simulink model "RB_KAIROS_impControl_repulsive"  (R2020b)
settings: Solver=ode4  StartTime=0.0  StopTime=t_end  FixedStep=Ts  RelTol=1e-3
values from neighbouring files (symbols this model uses):
  am = 0.3    [RB_KAIROS_ImpControl_OpSpace_quat_2020b_safety_main.m]
  am_r = 0.3    [RB_KAIROS_ImpControl_OpSpace_quat_2020b_safety_main.m]
  Kc = diag(50*ones(6,1))    [RB_KAIROS_ImpControl_OpSpace_quat_2020b_safety_main.m]
  Kp = 2*[400;400;400;400;0;0;0]    [RB_KAIROS_ImpControl_OpSpace_quat_2020b_safety_main.m]
  Kv = [1000;1000;1000;[300;300;300;300;300;300;300]]    [RB_KAIROS_ImpControl_OpSpace_quat_2020b_safety_main.m]
  model_sample_time = 0.001    [RB_KAIROS_ImpControl_OpSpace_quat_2020b_safety_main.m]
  q_dot_0 = zeros(10,1)    [RB_KAIROS_ImpControl_OpSpace_quat_2020b_safety_main.m]
  T_i = K    [RB_KAIROS_ImpControl_OpSpace_quat_2020b_safety_main.m]
  tau_ext = [0 0 0 0 0 0 0 0 0 0 0]    [RB_KAIROS_ImpControl_OpSpace_quat_2020b_safety_main.m]
  v_SMU = 10    [RB_KAIROS_ImpControl_OpSpace_quat_2020b_safety_main.m]
  vm = 0.5    [RB_KAIROS_ImpControl_OpSpace_quat_2020b_safety_main.m]
  vm_r = 0.5    [RB_KAIROS_ImpControl_OpSpace_quat_2020b_safety_main.m]
undefined symbols (not defined in the file or in its folder): DiscIntNeverNeededParam, magnitude, q_0, T_f
libraries: simulink x4, utils x4, transformations_lib x3
(part 12 of 17)

== matlab function RB_KAIROS_impControl_repulsive/Trajectory Generator/move2pose/fs_function ==
  data: opti_break output; T_est output; Tm input; time_step input; t input; vc input; vd input; vm input; v_smu input; am input; Gamma input; Theta input; k input; T_scale input; time_factor output; interpoly input; rethink_point input; start_lvl input; stop_lvl input; reset input
function [opti_break,T_est,time_factor] = fs_function_time_rethink(Tm, time_step, t, vc, vd, vm, v_smu, am, Gamma, Theta, k, T_scale, interpoly, rethink_point, start_lvl, stop_lvl, reset)
%%% This function decides which version to call; Or when/if a rethink is
%%% done.
% 0 =       internship version (only with minor bugfixes)
% 1 and 2 = start with half the velocity, then rethink, then linear part and
%           rest is the original full half
% 3 =       general solution, heading to vd always (best option)
% 4 =       general solution, heading to v_smu if going down

time_factor = 0;
opti_break = 0;
T_est = 0;
psi  = psi_velocity(vm, vd);
switch rethink_point
    case 0
        time_factor = fs_function_time_f(t, T_scale, psi, Gamma, Theta, k, interpoly);
    case 1
        T = T_calc(vc,vd,vm,am,T_scale,interpoly);
        [time_factor,opti_break,T_est] = fs_function_time_hlf(Tm, t, T, psi, Gamma, Theta, k, interpoly, time_step);
    case 2
        [time_factor,opti_break,T_est] = fs_function_time_g(Tm, t, T_scale, psi, Gamma, Theta, k, interpoly, time_step, 0, 0.5, 3, vm, am, v_smu, reset);
    case 3
        [time_factor,opti_break,T_est] = fs_function_time_g(Tm, t, T_scale, psi, Gamma, Theta, k, interpoly, time_step, start_lvl, stop_lvl, rethink_point, vm, am, v_smu, reset);
    case 4
        [time_factor,opti_break,T_est] = fs_function_time_g(Tm, t, T_scale, psi, Gamma, Theta, k, interpoly, time_step, start_lvl, stop_lvl, rethink_point, vm, am, v_smu, reset);
    otherwise
        error('Unknown rethink_point');       %rest
end

end

function [time_factor,opti_break,T_est] = fs_function_time_g(Tm, t, T_scale, psi, Gamma, Theta, k, interpoly, time_step, start_lvl, stop_lvl, rethink_point, vm, am, v_smu, reset)
%FS_FUNCTION_TIME computes the scaling factor for the next timestep. The idea is 
% similar to equotation (14) of the reference. This is
% achieved by the introduction of time t and setting a duration T for the
% adaption.
%
% This is the most general solution so far. It accelerates till am and then
% it stays on this level till it has to decelerate again to reach the new
% velocity level. The velocity level could be updated in any timestep.
%
% Reference:
% [1] S. Haddadin, A. Albu-Schäffer, A. De Luca, and G. Hirzinger, 
% "Collision detection and reaction: A contribution to safe physical 
% human-robot interaction,” International Conference on Intelligent Robots 
% and Systems, pp. 3356–3363, 2008.
%
% Input variables
% Tm          = Maximum time left for adaption
% t           = Current runtime
% T_scale     = Scaling factor for duration of adaption
% psi         = Scaling factor for time
% Gamma       = Optional dead-zone between stop and reverting motion (set 0
%               for deactivation)
% Theta       = Optional smoothness or strechting(set 1 for deactivation) 
% k           = speed factor for pushing back; 1=deactivated; the higher 
%               the faster the reverting motion
% interpoly   = Which interpolation to use
% time_step   = Duration of one time step
% start_lvl   = percentage for delta_psi_start: [0;1[ (Do not set to near to one!)
% stop_lvl    = percentage for delta_psi_stop: [0;1[ (Do not set to near to one!)
% rethink_point
%             = choose on which velocity the percentage is used
% vm          = maximum allowed velocity
% am          = maximum allowed acceleration
% v_smu       = Real v_smu
% reset       = If this is one, the psi_1 variable is reseted; only needed
%               due to reversing motion
%
% Output variables
% time_factor = Factor for scaling the next time increment; 0=Stop motion;
%               1= Normal speed; negative values = revert motion
% opti_break  = Trigger for optimal breaking; is set to 1 if Tm<T_est
% T_est       = Current estimate of the duration of the adaption motion


% In general variables with ..._1 belong to previous runs of the code and
% variables with numbers at the end belong to the corresponding phase. 
% Phase 1 is the start of an adaption motion. On this phase the
% acceleration is increased to am. In phase 2 the acceleration is constant
% on level am, which means that the velocity is linear. The decrease of the
% acceleration to zero again is called phase 3.
% A single i in the name of a varibale, means an inital value of something
% and the same holds for f for final value. m is maximum, d is desired.
% Small t is a absolut time, whereas capital T is a time duration.


%% Initialize persistent variables for adaption motion
persistent psi_1 adpt phase restart ti1 T1 psii1 psif1 ti2 T2 parameter2 ti3 T3 psii3 psif3 opti_break_mem psi_delta_start psi_delta_stop
if isempty(psi_1)
    psi_1 = psi;    %remembers the psi from last run
end
if isempty(adpt)
    adpt = false;   %stores if an adaption motion is activated
end
if isempty(phase)
    phase = 0;         %phase of adaption
end
if isempty(restart)
    restart = -1;         %At end of phase 3 the psi must be stored and restarts an adpation process
end
if isempty(ti1)
    ti1 = 0;         %Initial time step for phase 1
end
if isempty(T1)
    T1 = 0;         %Initial time duration phase 1
end
if isempty(psii1)
    psii1 = 0;      %Initial psi for phase 1
end
if isempty(psif1)
    psif1 = 0;         %final psi for phase 1
end
if isempty(ti2)
    ti2 = 0;         %Initial time step for phase 2
end
if isempty(T2)
    T2 = 0;         %duartion phase 2
end
if isempty(parameter2)
    parameter2 = zeros(2,1);         %Parameter of linear part / phase 2: p(2)*t + p(1)
end
if isempty(ti3)
    ti3 = 0;         %Initial time step for phase 3
end
if isempty(T3)
    T3 = 0;         %duration phase 3
end
if isempty(psii3)
    psii3 = 0;         %Initial psi for phase 3
end
if isempty(psif3)
    psif3 = 0;         %Initial psi for phase 3
end
if isempty(opti_break_mem)
    opti_break_mem = 0;         %memory of opti break; (holds trigger while adaption)
end
if isempty(psi_delta_start)
    psi_delta_start = 0;         %delta of velocity which the start of an adaption needs
end
if isempty(psi_delta_stop)
    psi_delta_stop = 0;         %delta of velocity which the stop of an adaption needs
end

T_est = 0; %init
psi_eps = 1e-6; %lowest psi difference an adaption starts; lower than in mogen, since psi is percentage of velocity

if reset==true %only needed because of reverting motion; if original start point is reached psi_1 has to be reseted to prevent errors at a restart.
    psi_1=0;
    adpt=false;
    restart = -1;
end

%% This If runs only for one timestep!!!
% If current psi is unequal to old one 
% Not directly at the beginning
% Dont start new while a adaption is still running, to prevent reset of
%   initial values
if psi~=psi_1 && t>time_step && adpt==false ...
        || restart>=0 && adpt==false
    
    if restart==psi %This if prevents a adaption if restart was set to the current vm (only possible with startoptions)
        adpt = false;
        phase = 0;
        restart = -1;
        
    % This if prevents adaptions if the difference in the desired velocity
    % is below the threshold psi_eps. To save the current velocity the
    % restart variable is used again. This also means that if the psi is
    % changing with a rate lower than the threshold, it is neccessary to
    % also compare the current velocity (in restart) and the current
    % desired velocity. If these two are more than the threshold it is
    % possible to adapt with the minimum adaption function.
    elseif (restart==-1 && abs(psi-psi_1)<psi_eps) ||...
           (restart>=0  && abs(psi-psi_1)<psi_eps && abs(psi-restart)<psi_eps)
        adpt = false; 
        phase = 0;
        if restart == -1 %For preventing a small error, because the psi has changed, while the non-adaption calculation
           restart = psi_1; 
        end
        
    else
        adpt=true;          % Activate adaption
        phase=1;            % start with phase 1
        ti1=t;               % Set initial timestep to current step
        
        %%% inital set of position, velo, acceleration for adaption motion
        if restart>=0
            psii1 = restart; 
        else
            psii1 = psi_1;
        end

        %%% Calc basic velocity levels
        psi_heading = psi; % init; psi_heading the velocity level the program is looking to, while calculating the v_deltas

        %For making sure that it is heading to v_smu always, while going down (Mazins way)
        if psi>psii1 && rethink_point == 4
            psi_smu  = psi_velocity(vm, v_smu);
            psi_heading = psi_smu; 
        end

        % velocity deltas at begin and end of adaption: 
        % mind the signs!!
        psi_delta_start = ((psi_heading-psii1)*(1-start_lvl))/2;
        psi_delta_stop  = ((psii1-psi_heading)*(1-stop_lvl))/2;

        %%% Calculation of Phase 1 and basic parameters
        
        %This is the final psi of the start / phase 1
        psif1 = psii1+2*psi_delta_start; 
        % Duration of adaption
        T1 = T_calc(psii1,psif1,vm,am,T_scale,interpoly);              
        if interpoly == 0
            adpt=false;         %no adatption  
            phase = 0;
        end

        %%% Phase 2
        ti2 = ti1+T1/2; % initial time of linear part
        
        %differentiate psi = maximum psi acceleration
        psii2   = adpt_fct(ti2,ti1,T1,psii1,psif1,interpoly);
        psii2_1 = adpt_fct(ti2-time_step,ti1,T1,psii1,psif1,interpoly);
        parameter2(2) = (psii2-psii2_1)/time_step;
        parameter2(1) = psii2;

        % reset variables
        restart = -1;
    end
end

%% Update function; runs always in phase 1 and phase 2 to update duration and check final levels
if adpt == true && (phase == 1 || phase == 2)
    
    %%% First decide to which velocity the program should go. This is
    %%% necessesary since the current vm could be higher than the velocity
    %%% level wich could be reached with an imdiate introduction of phase
    %%% 3. This nearest velocity level which can currently be reached is
    %%% called psi_near and calculated first   
    
    % evaluate linear part at last timestep
    t2 = t-ti2-time_step; 
    q2 = zeros(2,1); 
    q2(1) = parameter2(2)*t2+parameter2(1);
    q2(2) = parameter2(2);

    % Calculate nearest velocity psi_near
    if phase == 1
        % in phase 1 it is the start velocity plus both deltas, without
        % linear part
        psi_near = psii1+psi_delta_start-psi_delta_stop; %mind the signs!!!
    else
        % while linear part it is the current velocity level plus what is
        % needed to stop adaption.
        psi_near = q2(1)-psi_delta_stop; %mind the signs!!!
    end
    
    % this is now the decision to which velocity the update should go to
    if psii1>psif1 && psi>=psi_near
        psi_up = psi_near;
    elseif psii1<psif1 && psi<=psi_near
        psi_up = psi_near;
    else
        psi_up = psi;
    end 

    % calc final velocity of phase 2
    psif2 = psi_up+psi_delta_stop; %target minus stopping
    T2 = ((psif2-parameter2(1))/parameter2(2));% Exact Duration of phase 2

    % Parameters for Phase 3 = stopping adaption part
    ti3 = ti2 + T2; % initial time for phase 3

    % set virtual starting point of phase 3
    psii3 = psi_up+2*psi_delta_stop; 

    % Also set final value of phase 3
    psif3 = psi_up;

    % This not directly the duration of phase 3, because of the virtual part
    T3 = T_calc(psii3,psif3,vm,am,T_scale,interpoly);              % Duration of adaption
    
end

%% This If runs only for one timestep!!!
% Phase 1 => Phase 2
if phase == 1 && t>=ti2 %End of phase 1
    phase = 2;
end

%% This If runs only for one timestep!!!
% Phase 2 => Phase 3
if phase == 2 && t>=ti3 %End of phase 2
    phase = 3;
end

%% If adaption motion needed
if adpt == true 
    psi_adpt = 0; %init for simulink
    %%% calculate the adaption psi, which takes time from ti to
    % ti+T. t is the current runtime, _i initial values, _f final
    % values, _m maximum values
    if phase == 1
        %%% opti_break
        T_est = (T1/2+T2+T3/2)-(t-ti1);
        if Tm<T_est
            opti_break_mem = 1; 
        end
        psi_adpt = adpt_fct(t,ti1,T1,psii1,psif1,interpoly);
    elseif phase == 2
        %%% opti_break
        T_est = ((T2+T3/2)-(t-ti2));
        if Tm<T_est
            opti_break_mem = 1; 
        end
        psi_adpt = parameter2(2)*(t-ti2) + parameter2(1);
    elseif phase == 3
        %if time is equal than the finish time => adaption motion is complete
        %But it is aborted one timestep earlier, since the finish timestep
        %is already computed correctly by the standard interpolator.
        if t>=ti3+T3/2-1*time_step  
            adpt=false;     %If adaption finished => reset
            phase = 0;
            opti_break_mem = 0; % also reset opti break
            % Calculate finish time_step here because vm could be not equal
            % to final reached velocity level
            psi_adpt = psif3;
            if psi~=psif3  %If adaption is finished, but the vm value has changed again => restart from current velocity on
                restart = psif3;
            else
                restart = -1;
            end            
        else
            % opti_break
            T_est = T3/2-(t-ti3);
            if Tm<T_est
                opti_break_mem = 1; 
            end
        
            % Adaption to vm velocity
            tx = -T3/2; %exact time shift tx,  between ti3 and virtual start point of adaption in phase 3
            % Evaluate adaption function, shift with tx in time ...
            psi_adpt = adpt_fct(t,ti3+tx,T3,psii3,psif3,interpoly);
        end 
    end

    % This computes the time_factor with the standard fs_function, if there is
    % an adaption running
    if psi_adpt<0
        psi_adpt=0;
    end
    % Linear decline needed here, since smoothness is in time
    time_factor = fs_function_lin(psi_adpt, Gamma, Theta, k);

else %% time_factor without adaption  
    % This computes the time_factor with the standard fs_function, if there is
    % no adaption
    time_factor = fs_function_lin(psi, Gamma, Theta, k);
end

opti_break = opti_break_mem;
psi_1 = psi;  %remember current psi

end

function [time_factor,opti_break,T_est] = fs_function_time_hlf(Tm, t, T, psi, Gamma, Theta, k, interpoly, time_step)
%FS_FUNCTION_TIME computes the scaling factor for the next timestep. The idea is 
% similar to equotation (14) of the reference, except that Theta adds a
% parameter for smoother decline and it allows a slower decline. This is
% achieved by the introduction of time t and setting a duration T for the
% adaption. Phi function underneath is similar to (16) of the reference.
%
% This is the more adaptive version which rethinks about the target
% velocity after the maximum acceleration is reached. And also it is
% allowed to change the velocity reference while an adaption is running.
%
% Reference:
% [1] S. Haddadin, A. Albu-Schäffer, A. De Luca, and G. Hirzinger, 
% "Collision detection and reaction: A contribution to safe physical 
% human-robot interaction,” International Conference on Intelligent Robots 
% and Systems, pp. 3356–3363, 2008.
%
% Input variables
% Tm          = Maximum time left for adaption
% t           = Current runtime
% T           = Duration of adaption
% psi         = Scaling factor for time; 0=No scaling; Theta=stop;
%               >Theta+Gamma = revert motion
% Gamma       = Optional dead-zone between stop and reverting motion (set 0
%               for deactivation)
% Theta       = Optional smoothness or strechting(set 1 for deactivation) 
% k           = speed factor for pushing back; 1=deactivated; the higher 
%               the faster the reverting motion
% interpoly   = Which interpolation to use
% time_step   = Duration of one time step
%
% Output variables
% time_factor = Factor for scaling the next time increment; 0=Stop motion;
%               1= Normal speed; negative values = revert motion
% opti_break  = Trigger for optimal breaking; is set to 1 if Tm<T_est
% T_est       = Current estimate of the duration of the adaption motion
    
%% Initialize persistent variables for adaption motion
persistent psi_1 adpt ti psi_i Tf psif psi_up phase dpsi_m Tx T_up psi_restart opti_break_mem
if isempty(psi_1)
    psi_1 = psi;    %remembers the psi from last run
end
if isempty(adpt)
    adpt = false;   %stores if an adaption motion is activated
end
if isempty(ti)
    ti = 0;         %Initial time step for adaption motion
end
if isempty(psi_i)
    psi_i = 0;      %Initial psi for adaption motion
end
if isempty(Tf)
    Tf = 0;         %Initial time duration for adaption motion
end
if isempty(psif)
    psif = 0;         %Initial final psi
end
if isempty(psi_up)
    psi_up = 0;         %Update psi, after rethink
end
if isempty(phase)
    phase = 0;         %phase of adaption
end
if isempty(dpsi_m)
    dpsi_m = 0;         %maximum of psi dot; slope of phase 2
end
if isempty(Tx)
    Tx = 0;         %End of phase 2 == Middle of initial adaption reached
end
if isempty(T_up)
    T_up = 0;         %Update duration, after rethink
end
if isempty(psi_restart)
    psi_restart = -1;         %At end of phase 4 the psi must be stored and restarts an adpation process
end
if isempty(opti_break_mem)
    opti_break_mem = 0;         %memory of opti break; (holds trigger while adaption)
end
T_est = 0; %init

%% This If runs only for one timestep!!!
% If current psi is unequal to old one 
% Not directly at the beginning
% Dont start new while a adaption is still running, to prevent reset of
%   initial values
if abs(psi-psi_1)>1e-6 && t>time_step && adpt==false ...
        || psi_restart>=0 && adpt==false
    adpt=true;          % Activate adaption
    phase=1;            % start with phase 1
    ti=t;               % Set initial timestep to current step
    psif = psi;         % final value is new psi
    Tf=T;               % Duration of adaption
    %%% inital set of position, velo, acceleration for adaption motion
    if psi_restart>=0
        psi_i = psi_restart; 
    else
        psi_i = psi_1;
    end

    if interpoly == 0
        adpt=false;         %no adatption  
    end
    
    %%% Phase 2
    %differentiate current psi = maximum acceleration
    psi_current   = adpt_fct(ti+Tf/4,ti,Tf/2,psi_i,0.5*(psi_i+psif),interpoly);
    psi_current_1 = adpt_fct(ti+Tf/4,ti+time_step,Tf/2,psi_i,0.5*(psi_i+psif),interpoly);
    dpsi_m = (psi_current-psi_current_1)/time_step;
    psi_up = psif; % Save current psi as update (update stuff was intended to update final values while rethink, but is not working)
    T_up = Tf; % Duration of adaption 
    shift = 0.25*(3*psi_i+psif)-dpsi_m*Tf/4;  % shift for linear part
    Tx = (0.5*(psi_i+psi_up)-shift)/dpsi_m;     % End of linear part
        
    % reset variables
    psi_restart = -1;
    
end

%% This If runs only for one timestep!!!
% Rethink?!
if phase == 1 && t>=ti+Tf/4 %End of phase 1
    if psi_i<psif && psi<=0.5*(psi_i+psif) % If human stops or goes away meanwhile
        phase = 4;
    elseif psi_i>psif && psi>=0.5*(psi_i+psif) % If human stops or goes away meanwhile
        phase = 4;
    else
        phase = 2;
    end
end

%% This If runs only for one timestep!!!
% phase 2 => phase 3
if phase == 2 && t>=ti+Tx+time_step %End of phase 2
    phase = 3;
end

%% If adaption motion needed
if adpt == true 
    psi_adpt = 0; %init for simulink
    %%% calculate the adaption psi, which takes time from ti to
    % ti+T. t is the current runtime, _i initial values, _f final
    % values, _m maximum values
    if phase == 1
        %%% opti_break
        T_est = ((Tf/2+Tx)-(t-ti));
        if Tm<T_est
            opti_break_mem = 1; 
        end
        psi_adpt = adpt_fct(t,ti,Tf/2,psi_i,0.5*(psi_i+psif),interpoly);
    elseif phase == 2
        %%% opti_break
        T_est = ((Tf/2+Tx)-(t-ti));
        if Tm<T_est
            opti_break_mem = 1; 
        end
        shift = 0.25*(3*psi_i+psif)-dpsi_m*Tf/4;
        psi_adpt = dpsi_m * (t-ti) + shift;
    elseif phase == 3
        %%% opti_break
        T_est = ((Tf/2+Tx)-(t-ti));
        if Tm<T_est
            opti_break_mem = 1; 
        end
        tx = (T_up/2)-Tx;
        psi_adpt = adpt_fct(t,ti-tx,T_up,psi_i,psi_up,interpoly);
        %if time is equal than the finish time => adaption motion is complete
        %But it is aborted one timestep earlier, since the finish timestep
        %is already computed correctly by the standard interpolator.
        if t>=(ti+T_up-tx-1*time_step)  
            adpt=false;     %If adaption finished => reset
            phase = 0;
            opti_break_mem = 0; 
            if psi~=psi_up  %If adaption is finished, but the psi value has changed again => restart from current psi on
                psi_restart = psi_up;
            else
                psi_restart = -1;
            end
        end
    elseif phase == 4
        %%% opti_break
        T_est = ((0.25*Tf)-(t-(ti+Tf/4)));
        if Tm<T_est
            opti_break_mem = 1; 
        end
        
        psi_adpt = adpt_fct(t,ti,Tf/2,psi_i,0.5*(psi_i+psif),interpoly);
        %if time is equal than the finish time => adaption motion is complete
        %But it is aborted one timestep earlier, since the finish timestep
        %is already computed correctly by the standard interpolator.
        if t>=(ti+Tf/2-1*time_step)  
            adpt=false;     %If adaption finished => reset
            phase = 0;
            opti_break_mem = 0; 
            psi_restart = 0.5*(psi_i+psif);
        end

    end

    % This computes the time_factor with the standard fs_function, if there is
    % an adaption running
    if psi_adpt<0
        psi_adpt=0;
    end
    time_factor = fs_function_lin(psi_adpt, Gamma, Theta, k);

else %% time_factor without adaption  
    % This computes the time_factor with the standard fs_function, if there is
    % no adaption
    % Linear decline needed here, since smoothness is in time
    time_factor = fs_function_lin(psi, Gamma, Theta, k);
end

opti_break = opti_break_mem;
psi_1 = psi;  %remember current psi

end

function time_factor = fs_function_time_f(t, T, psi, Gamma, Theta, k, interpoly)
%FS_FUNCTION_TIME computes the scaling factor for the next timestep. It is 
% similar to equotation (14) of the reference, except that Theta adds a
% parameter for smoother decline and it allows a slower decline. This is
% achieved by the introduction of time t and setting a duration T for the
% adaption. Phi function underneath is similar to (16) of the reference.
%
% Reference:
% [1] S. Haddadin, A. Albu-Schäffer, A. De Luca, and G. Hirzinger, 
% "Collision detection and reaction: A contribution to safe physical 
% human-robot interaction,” International Conference on Intelligent Robots 
% and Systems, pp. 3356–3363, 2008.
%
% Input variables
% t           = Current runtime
% T           = Duration of adaption
% psi         = Scaling factor for time; 0=No scaling; Theta=stop;
%               >Theta+Gamma = revert motion
% Gamma       = Optional dead-zone between stop and reverting motion (set 0
%               for deactivation)
% Theta       = Optional smoothness or strechting(set 1 for deactivation) 
% k           = speed factor for pushing back; 1=deactivated; the higher 
%               the faster the reverting motion
% interpoly   = Which interpolation to use
%
% Output variables
% time_factor = Factor for scaling the next time increment; 0=Stop motion;
%               1= Normal speed; negative values = revert motion
    
%% Initialize persistent variables for adaption motion
persistent psi_1 adpt ti psi_i
if isempty(psi_1)
    psi_1 = psi;    %remembers the psi from last run
end
if isempty(adpt)
    adpt = false;   %stores if an adaption motion is activated
end
if isempty(ti)
    ti = 0;         %Initial time step for adaption motion
end
if isempty(psi_i)
    psi_i = 0;      %Initial psi for adaption motion
end

% needed to delay tanhlog with one timestep
tanhlog_delay = 0;

%% This If runs only for one timestep!!!
% If current psi is unequal to old one 
% Not directly at the beginning
% Dont start new while a adaption is still running, to prevent reset of
%   initial values
if abs(psi-psi_1)>1e-6 && t>0.001 && adpt==false                          
    adpt=true;          % Activate adaption
    ti=t;               % Set initial timestep to current step

    %%% inital set of position, velo, acceleration for adaption motion 
    psi_i = psi_1;
    tanhlog_delay = 1;    
end

%% If adaption motion needed
if adpt == true 

    %%% calculate the adaption psi, which takes time from ti to
    % ti+T. t is the current runtime, _i initial values, _f final
    % values, _m maximum values

    switch interpoly
        case 0
            adpt=false;         %no adatption  
            psi_adpt = psi;
        case 1
            if tanhlog_delay == 1
                psi_adpt = psi_i;
                tanhlog_delay = 0;
            else
                psi_adpt = tanhlog(t-ti,T,psi_i,psi);  %tanhlog
            end
        case 2
            psi_adpt = cosine(t-ti,T,psi_i,psi);   %Cosine version
        case 3
            psi_adpt = poly3(t-ti,T,psi_i,psi);    %poly3
        case 4
            psi_adpt = poly4(t-ti,T,psi_i,psi);    %poly4
        case 5
            psi_adpt = poly5(t-ti,T,psi_i,psi);    %poly5 
        case 6
            psi_adpt = poly6(t-ti,T,psi_i,psi);    %poly6 
        case 7
            psi_adpt = poly7(t-ti,T,psi_i,psi);    %poly7
        case 10
            psi_adpt = tanhmean(t-ti,T,psi_i,psi);    %tanhmean 
        otherwise
            error('Unknown adaption motion');   %rest
    end

    % This computes the time_factor with the standard fs_function, if there is
    % an adaption running
    time_factor = fs_function_lin(psi_adpt, Gamma, Theta, k);

    %if time is equal than the finish time => adaption motion is complete
    %But it is aborted one timestep earlier, since the finish timestep
    %is already computed correctly by the standard interpolator.
    if t>=(ti+T-0.001)  
        adpt=false;     %If adaption finished => reset
    end
    
else %% time_factor without adaption  
    % This computes the time_factor with the standard fs_function, if there is
    % no adaption
    % Linear decline needed here, since smoothness is in time
    time_factor = fs_function_lin(psi, Gamma, Theta, k);
end

psi_1 = psi;  %remember current psi

end

function [psi_adpt] = adpt_fct(t,ti,T,psi_i,psi,interpoly)

    
    %%% calculate the adaption psi, which takes time from ti to
    % ti+T. t is the current runtime, _i initial values, _f final
    % values, _m maximum values
    
    switch interpoly
        case 0
            psi_adpt = psi;                        %no adaption
        case 1
            psi_adpt = tanhlog(t-ti,T,psi_i,psi);  %tanhlog
        case 2
            psi_adpt = cosine(t-ti,T,psi_i,psi);   %Cosine version
        case 3
            psi_adpt = poly3(t-ti,T,psi_i,psi);    %poly3
        case 4
            psi_adpt = poly4(t-ti,T,psi_i,psi);    %poly4
        case 5
            psi_adpt = poly5(t-ti,T,psi_i,psi);    %poly5 
        case 6
            psi_adpt = poly6(t-ti,T,psi_i,psi);    %poly6 
        case 7
            psi_adpt = poly7(t-ti,T,psi_i,psi);    %poly7
        case 10
            psi_adpt = tanhmean(t-ti,T,psi_i,psi); %tanhmean 
        otherwise
            error('Unknown adaption motion');      %rest
    end
    
end

function [T] = T_calc(psi_start,psi_goal,vm,am,T_scale,interpoly)

    %%% Duration of adaption motion
    T_standard = ((abs(psi_start-psi_goal)*vm)/am);

    switch interpoly
        case 1
            T = T_standard*2;       %tanhlog
        case 2
            T = T_standard*1.57;    %Cosine version
        case 3
            T = T_standard*1.5;     %poly3
        case 4
            T = T_standard*1.78;    %poly4
        case 5
            T = T_standard*1.87;    %poly5
        case 6
            T = T_standard*2.03;    %poly6
        case 7
            T = T_standard*2.18;    %poly7 
        case 10
            T = T_standard*1.99;    %tanhmean 
        otherwise
            T = T_standard*2;       %rest
    end

    % Scale Duration if needed
    T = T*T_scale;

end

function time_factor = fs_function(psi, Gamma, Theta, k)
%FS_FUNCTION computes the scaling factor for the next timestep. It is 
% similar to equotation (14) of the reference, except that Theta adds a
% parameter for smoother decline. Phi function underneath is similar to
% (16) of the reference.
%
% Reference:
% [1] S. Haddadin, A. Albu-Schäffer, A. De Luca, and G. Hirzinger, 
% "Collision detection and reaction: A contribution to safe physical 
% human-robot interaction,” International Conference on Intelligent Robots 
% and Systems, pp. 3356–3363, 2008.

% Input variables
% psi         = Scaling factor for time; 0=No scaling; Theta=stop;
%               >Theta+Gamma = revert motion
% Gamma       = Optional dead-zone between stop and reverting motion (set 0
%               for deactivation)
% Theta       = Optional smoothness or strechting(set 1 for deactivation) 
% k           = speed factor for pushing back; 1=deactivated; the higher 
%               the faster the reverting motion

% Output variables
% time_factor = Factor for scaling the next time increment; 0=Stop motion;
%               1= Normal speed; negative values = revert motion
       
time_factor = 0;
if 0 <= psi && psi < Theta    %Equ. (14)
    time_factor = phi(psi, Theta);
elseif Theta <= psi && psi <= Theta+Gamma
    time_factor = 0;
elseif Theta+Gamma < psi && psi <= 2*Theta+Gamma
    time_factor = k*phi(psi-Theta-Gamma, Theta)-k;
elseif 2*Theta+Gamma < psi
    time_factor = -k;
else
    error('Trajectory scaling - fs_function: psi wrong (e.g. psi<0)');
end

end

function [psi_smooth] = phi(psi, Theta)
%PHI computes formular (16); smoother decline of factor
%
% Reference:
% [1] S. Haddadin, A. Albu-Schäffer, A. De Luca, and G. Hirzinger, 
% "Collision detection and reaction: A contribution to safe physical 
% human-robot interaction,” International Conference on Intelligent Robots 
% and Systems, pp. 3356–3363, 2008.
%
% Input variables
% psi     = Scaling factor for time (could be vector to here)
% Theta   = Optional smoothness or strechting(set 1 for deactivation)
%
% Output variables
% psi_smooth = smoother psi value

psi_smooth = 0.5.*(ones(size(psi))+cos((1/Theta)*pi.*psi)); %Equ. (16)

end

function time_factor = fs_function_lin(psi, Gamma, Theta, k)
%FS_FUNCTION_LIN computes the scaling factor for the next timestep. It is 
% similar to equotation (14) of the reference, except that Theta adds a
% parameter for smoother decline. Phi function underneath is linear decline
%
% Reference:
% [1] S. Haddadin, A. Albu-Schäffer, A. De Luca, and G. Hirzinger, 
% "Collision detection and reaction: A contribution to safe physical 
% human-robot interaction,” International Conference on Intelligent Robots 
% and Systems, pp. 3356–3363, 2008.

% Input variables
% psi         = Scaling factor for time; 0=No scaling; Theta=stop;
%               >Theta+Gamma = revert motion
% Gamma       = Optional dead-zone between stop and reverting motion (set 0
%               for deactivation)
% Theta       = Optional smoothness or strechting(set 1 for deactivation) 
% k           = speed factor for pushing back; 1=deactivated; the higher 
%               the faster the reverting motion

% Output variables
% time_factor = Factor for scaling the next time increment; 0=Stop motion;
%               1= Normal speed; negative values = revert motion
       
time_factor = 0;
if 0 <= psi && psi < Theta    %Equ. (14)
    time_factor = lin(psi, Theta);
elseif Theta <= psi && psi <= Theta+Gamma
    time_factor = 0;
elseif Theta+Gamma < psi && psi <= 2*Theta+Gamma
    time_factor = k*lin(psi-Theta-Gamma, Theta)-k;
elseif 2*Theta+Gamma < psi
    time_factor = -k;
else
    error('Trajectory scaling - fs_function: psi wrong (e.g. psi<0)');
end

end

function [psi_smooth] = lin(psi, Theta)
%LIN computes linear decline of factor. selfmade
%
% Input variables
% psi     = Scaling factor for time (could be vector to here)
% Theta   = Optional smoothness or strechting(set 1 for deactivation)
%
% Output variables
% psi_smooth = smoother psi value

psi_smooth = 1-(psi/Theta);

end

function [psi] = tanhlog_old(t,T,psi_i,psi_f)
%TANHLOG computes a 2 tanh-log trajectories between initial (_i) 
%values and final (_f) values of psi. The first goes to a virtual line in 
%the middle and the second back to d_psi_f=0.
%taken from Internet

psi_mean = (psi_f+psi_i)/2;             % calculate mean value of inital and final value
virt_slope = (4*psi_mean-4*psi_i)/T;    % define slope of virtual line 
virt_shift = psi_mean - virt_slope*T/2; % compute the shift of the virtual line

if t<=T/2 %first part for inital to virtual
    a = 0;         
    b = psi_i; 
    c = virt_slope;
    d = virt_shift;
    k = d-b;

    x = (a*t+b-c*t-d+k)/(2*k);
    w = (tanh(((log(1-x))^2-(log(x))^2)/3)+1)/2;
    p = tanh((log(2-x)-log(x))*(1-(1/sqrt(2))*(log(2-x)+log(x))))+2*x-1;
    q = tanh((log(x+1)-log(1-x))*(1-(1/sqrt(2))*(log(1-x)+log(x+1))));
    s = p*(1-w)+q*w;

    psi = k*s+c*t+d-k;
else    %second part from virtual to final
    a = virt_slope;
    b = virt_shift;
    c = 0;     
    d = psi_f; 
    k = (d-b)*(1/3); %k has to be computed a bit different. Math...

    x = (a*t+b-c*t-d+k)/(2*k);
    w = (tanh(((log(1-x))^2-(log(x))^2)/3)+1)/2;
    p = tanh((log(2-x)-log(x))*(1-(1/sqrt(2))*(log(2-x)+log(x))))+2*x-1;
    q = tanh((log(x+1)-log(1-x))*(1-(1/sqrt(2))*(log(1-x)+log(x+1))));
    s = p*(1-w)+q*w;

    psi = k*s+c*t+d-k;
end

end

function [psi] = tanhlog(t,T,psi_i,psi_f)
%TANHLOG computes a 2 tanh-log trajectories between initial (_i) 
%values and final (_f) values of psi. The first goes to a virtual line in 
%the middle and the second back to d_psi_f=0.
%taken from Internet

% Threshold for checks
th = 1e-6;

psi_mean = (psi_f+psi_i)/2;             % calculate mean value of inital and final value
virt_slope = (4*psi_mean-4*psi_i)/T;    % define slope of virtual line 
virt_shift = psi_mean - virt_slope*T/2; % compute the shift of the virtual line

% tanhlog cannot compute first and last value, due to ln(0) problems.
% So if tanhlog is evaluated around zero and below, psi_i is returned.
% And if tanhlog is evaluated at a time near or higher than the planned
% duration psi_f is returned.
if t<th
    psi = psi_i;
elseif T-t<th
    psi = psi_f;
else
    if t<=T/2 %first part for inital to virtual
        a = 0;         
        b = psi_i; 
        c = virt_slope;
        d = virt_shift;
        k = d-b;
% 
%         if abs(k)>th
            x = (a*t+b-c*t-d+k)/(2*k);
%             if x>th && x<(1-th)
                w = (tanh(((log(1-x))^2-(log(x))^2)/3)+1)/2;
                p = tanh((log(2-x)-log(x))*(1-(1/sqrt(2))*(log(2-x)+log(x))))+2*x-1;
                q = tanh((log(x+1)-log(1-x))*(1-(1/sqrt(2))*(log(1-x)+log(x+1))));
                s = p*(1-w)+q*w;

                psi = k*s+c*t+d-k;
%             else 
%                 psi = 0;
%             end
%         else
%             psi = 0;
%         end
    else    %second part from virtual to final
        a = virt_slope;
        b = virt_shift;
        c = 0;     
        d = psi_f; 
        k = (d-b)*(1/3); %k has to be computed a bit different. Math...

%         if abs(k)>th
            x = (a*t+b-c*t-d+k)/(2*k);
%             if x>th && x<(1-th)
                w = (tanh(((log(1-x))^2-(log(x))^2)/3)+1)/2;
                p = tanh((log(2-x)-log(x))*(1-(1/sqrt(2))*(log(2-x)+log(x))))+2*x-1;
                q = tanh((log(x+1)-log(1-x))*(1-(1/sqrt(2))*(log(1-x)+log(x+1))));
                s = p*(1-w)+q*w;

                psi = k*s+c*t+d-k;
%             else 
%                 psi = 0;
%             end
%         else
%             psi = 0;
%         end
    end
end

end

function [psi] = cosine(t,T,psi_i,psi_f)
%COSINE computes a cosine trajectory between initial (_i) 
%values and final (_f) values of psi. t is the time since ti; T the
%duration
   
psi = 0.5*(psi_i+psi_f) + 0.5*(psi_i-psi_f)*cos((pi/T)*t);

end

function [psi] = poly3(t,T,psi_i,psi_f)
%POLY3 computes a polynomial trajectory of degree 3 between initial (_i) 
%values and final (_f) values of psi. selfmade with poly_calc

d_psi_i = 0; %with poly3 an adaption to the velocity of the change of psi would be possible
d_psi_f = 0;

a = [...
 conj(psi_i)
 conj(d_psi_i)
 (3*conj(psi_f))/T^2 - (2*conj(d_psi_i))/T - conj(d_psi_f)/T - (3*conj(psi_i))/T^2
 conj(d_psi_f)/T^2 + conj(d_psi_i)/T^2 - (2*conj(psi_f))/T^3 + (2*conj(psi_i))/T^3];

psi = a(1)+a(2)*t+a(3)*t^2+a(4)*t^3;

end

function [psi] = poly4(t,T,psi_i,psi_f)
%POLY4 computes a polynomial trajectory of degree 4 between initial (_i) 
%values and final (_f) values of psi. selfmade with poly_calc

d_psi_i = 0; %with poly4 an adaption to the velocity of the change of psi would be possible
d_psi_f = 0;
dd_psi_f = 0;

a = [...
                                                                                                    conj(psi_i)
                                                                                                  conj(d_psi_i)
       conj(dd_psi_f)/2 - (3*conj(d_psi_f))/T - (3*conj(d_psi_i))/T + (6*conj(psi_f))/T^2 - (6*conj(psi_i))/T^2
   (5*conj(d_psi_f))/T^2 + (3*conj(d_psi_i))/T^2 - conj(dd_psi_f)/T - (8*conj(psi_f))/T^3 + (8*conj(psi_i))/T^3
 conj(dd_psi_f)/(2*T^2) - conj(d_psi_i)/T^3 - (2*conj(d_psi_f))/T^3 + (3*conj(psi_f))/T^4 - (3*conj(psi_i))/T^4];

psi = a(1)+a(2)*t+a(3)*t^2+a(4)*t^3+a(5)*t^4;

end

function [psi] = poly5(t,T,psi_i,psi_f)
%POLY4 computes a polynomial trajectory of degree 4 between initial (_i) 
%values and final (_f) values of psi. selfmade with poly_calc

d_psi_i = 0; %with poly4 an adaption to the velocity of the change of psi would be possible
d_psi_f = 0;
dd_psi_i = 0;
dd_psi_f = 0;

a = [...
                                                                                                                                   conj(psi_i)
                                                                                                                                 conj(d_psi_i)
                                                                                                                              conj(dd_psi_i)/2
 conj(dd_psi_f)/(2*T) - (6*conj(d_psi_i))/T^2 - (4*conj(d_psi_f))/T^2 - (3*conj(dd_psi_i))/(2*T) + (10*conj(psi_f))/T^3 - (10*conj(psi_i))/T^3
 (7*conj(d_psi_f))/T^3 + (8*conj(d_psi_i))/T^3 - conj(dd_psi_f)/T^2 + (3*conj(dd_psi_i))/(2*T^2) - (15*conj(psi_f))/T^4 + (15*conj(psi_i))/T^4
   conj(dd_psi_f)/(2*T^3) - (3*conj(d_psi_i))/T^4 - (3*conj(d_psi_f))/T^4 - conj(dd_psi_i)/(2*T^3) + (6*conj(psi_f))/T^5 - (6*conj(psi_i))/T^5];

psi = a(1)+a(2)*t+a(3)*t^2+a(4)*t^3+a(5)*t^4+a(6)*t^5;

end

function [psi] = poly6(t,T,psi_i,psi_f)
%POLY6 computes a polynomial trajectory of degree 6 between initial (_i) 
%values and final (_f) values of psi. j_m is max jerk. selfmade with poly_calc

d_psi_i = 0; %with poly4 an adaption to the velocity of the change of psi would be possible
d_psi_f = 0;
dd_psi_i = 0;
dd_psi_f = 0;
j_m = 50;

a = [...
                                                                                                                                                           conj(psi_i)
                                                                                                                                                         conj(d_psi_i)
                                                                                                                                                      conj(dd_psi_i)/2
                                                                                                                                                           conj(j_m)/6
      conj(dd_psi_f)/(2*T^2) - (10*conj(d_psi_i))/T^3 - (5*conj(d_psi_f))/T^3 - (3*conj(dd_psi_i))/T^2 - conj(j_m)/(2*T) + (15*conj(psi_f))/T^4 - (15*conj(psi_i))/T^4
        (9*conj(d_psi_f))/T^4 + (15*conj(d_psi_i))/T^4 - conj(dd_psi_f)/T^3 + (4*conj(dd_psi_i))/T^3 + conj(j_m)/(2*T^2) - (24*conj(psi_f))/T^5 + (24*conj(psi_i))/T^5
 conj(dd_psi_f)/(2*T^4) - (6*conj(d_psi_i))/T^5 - (4*conj(d_psi_f))/T^5 - (3*conj(dd_psi_i))/(2*T^4) - conj(j_m)/(6*T^3) + (10*conj(psi_f))/T^6 - (10*conj(psi_i))/T^6];

psi = a(1)+a(2)*t+a(3)*t^2+a(4)*t^3+a(5)*t^4+a(6)*t^5+a(7)*t^6;

end

function [psi] = poly7(t,T,psi_i,psi_f)
%POLY6 computes a polynomial trajectory of degree 6 between initial (_i) 
%values and final (_f) values of psi. j_m is max jerk. selfmade with poly_calc

d_psi_i = 0; %with poly4 an adaption to the velocity of the change of psi would be possible
d_psi_f = 0;
dd_psi_i = 0;
dd_psi_f = 0;
ddd_psi_i = 0;
ddd_psi_f = 0;

a = [...
                                                                                                                                                                                                       conj(psi_i)
                                                                                                                                                                                                     conj(d_psi_i)
                                                                                                                                                                                                  conj(dd_psi_i)/2
                                                                                                                                                                                                 conj(ddd_psi_i)/6
           (5*conj(dd_psi_f))/(2*T^2) - (20*conj(d_psi_i))/T^3 - (15*conj(d_psi_f))/T^3 - (5*conj(dd_psi_i))/T^2 - conj(ddd_psi_f)/(6*T) - (2*conj(ddd_psi_i))/(3*T) + (35*conj(psi_f))/T^4 - (35*conj(psi_i))/T^4
                  (39*conj(d_psi_f))/T^4 + (45*conj(d_psi_i))/T^4 - (7*conj(dd_psi_f))/T^3 + (10*conj(dd_psi_i))/T^3 + conj(ddd_psi_f)/(2*T^2) + conj(ddd_psi_i)/T^2 - (84*conj(psi_f))/T^5 + (84*conj(psi_i))/T^5
 (13*conj(dd_psi_f))/(2*T^4) - (36*conj(d_psi_i))/T^5 - (34*conj(d_psi_f))/T^5 - (15*conj(dd_psi_i))/(2*T^4) - conj(ddd_psi_f)/(2*T^3) - (2*conj(ddd_psi_i))/(3*T^3) + (70*conj(psi_f))/T^6 - (70*conj(psi_i))/T^6
               (10*conj(d_psi_f))/T^6 + (10*conj(d_psi_i))/T^6 - (2*conj(dd_psi_f))/T^5 + (2*conj(dd_psi_i))/T^5 + conj(ddd_psi_f)/(6*T^4) + conj(ddd_psi_i)/(6*T^4) - (20*conj(psi_f))/T^7 + (20*conj(psi_i))/T^7];

psi = a(1)+a(2)*t+a(3)*t^2+a(4)*t^3+a(5)*t^4+a(6)*t^5+a(7)*t^6+a(8)*t^7;

end

function [psi] = tanhmean(t,T,psi_i,psi_f)
%TANHMEAN computes a tanh trajectory between initial (_i) 
%values and final (_f) values of psi. theta is the slope of the transition
%selfmade
                     
t_norm = t/T; %Normalized time necessary for this function
theta = 4;

psi = 0.5*(psi_i+psi_f) + 0.5*(psi_f-psi_i)*tanh(theta*(t_norm-0.5));

end

function psi  = psi_velocity(v_desired, v_safe)
%PSI_VELOCITY Computes a psi value from the comparison of two
%velocities. v_desired is the velocity the robot should move and v_safe
%sets an upper limit. The returned psi value scales down the velocity to a 
%safe value. Both values can be vectors, then the function checks the psi
%value for each dimension and returns the most restrictive psi (=highest).
%
% Input variables
% v_desired = The velocity the robot should move with
% v_safe    = The maximal velocity which is safe for this movement
%
% Output variables
% psi       = value for influencing the speed of the robot

psi = 0;
n = size(v_desired,2);  %n= dimension of velocity
psis = zeros(n,1);      %predefine vector for each dimension
for i=1:n               %Check each dimension
    psis(i) = psi_velocity_single(v_desired(i), v_safe(i));
end

psi = max(psis);        %Take most restrictive psi for all dimensions

end

function [psi_single] = psi_velocity_single(v_desired, v_safe)
%PSI_VELOCITY_SINGLE Computes a psi value from the comparison of two
%velocities. v_desired is the velocity the robot should move and v_safe
%sets an upper limit. The returned psi value scales down the velocity to a 
%safe value, if v_desired is greater than v_safe. This function compares
%only one dimension.
%
% Input variables
% v_desired  = The velocity the robot should move with
% v_safe     = The maximal velocity which is safe for this movement
%
% Output variables
% psi_single = value for influencing the speed of the robot

psi_single = 0;
if v_desired <= v_safe                   %No danger
    psi_single = 0;                     %=> No scaling
elseif v_desired > v_safe              %Desired velocity is dangerous
	psi_single = (1-(v_safe/v_desired));%=> Scaling of time to safe velocity
end

end

== matlab function RB_KAIROS_impControl_repulsive/EE to task space quaternion quantities/MATLAB Function3 ==
  data: qt_err input; qt_err_smaller_path output
function qt_err_smaller_path = fcn(qt_err)

if(qt_err(1) < 0)
    qt_err_smaller_path = -qt_err;
else
    qt_err_smaller_path = qt_err;
end

== matlab function RB_KAIROS_impControl_repulsive/CONTROLLER /MATLAB Function3 ==
  data: A input; A_lin output
function A_lin = eliminate_couplings(A)

A_lin = zeros(10,10);
A_lin(1:3,1:3) = A(1:3,1:3);
A_lin(4:10,4:10) = A(4:10,4:10);

end

== matlab function RB_KAIROS_impControl_repulsive/RB-KAIROS/Configuration space dynamics ==
  data: M input; q_ddot output; C input; g input; tau_ext input; tau input; q_dot input
function q_ddot = Config_space_dynamics(M,C,g,tau_ext,tau,q_dot)

q_ddot = M\(tau + tau_ext - C*q_dot - g);

== matlab function RB_KAIROS_impControl_repulsive/Trajectory Generator/MATLAB Function1 ==
  data: u input; y output
function y = euler_to_rotmatrix(u)

y = eul2rotm(u', 'XYZ');

== matlab function RB_KAIROS_impControl_repulsive/Trajectory Generator/MATLAB Function2 ==
  data: rpy input; omega output; rpyD input
% function omega = eul2omega(Phi, dPhi)
% 
% %XYZ
% omega = [cos(Phi(2))*cos(Phi(3)) sin(Phi(3)) 0;
%          -cos(Phi(2))*sin(Phi(3)) cos(Phi(3)) 0;
%          sin(Phi(2)) 0 1]*dPhi;
% 
% % ZYX
% % omega = [1 0 -sin(Phi(2));
% %          0 cos(Phi(3)) sin(Phi(3))*cos(Phi(2));
% %          0 -sin(Phi(3)) cos(Phi(3))*cos(Phi(2))]*dPhi;

function omega = eulxyzD2omega(rpy, rpyD)
%% Init
%#codegen
%$cgargs {zeros(3,1),zeros(3,1)}
assert(all(size(rpy) == [3 1]) && isreal(rpy), ...
  'eulxyzD2omega: rpy angles have to be [3x1] (double)'); 
assert(all(size(rpyD) == [3 1]) && isreal(rpyD), ...
  'eulxyzD2omega: rpy angles time derivatives have to be [3x1] (double)'); 

alpha_s = rpy(1);
beta_s = rpy(2);
gamma_s = rpy(3);

alphaD_s = rpyD(1);
betaD_s = rpyD(2);
gammaD_s = rpyD(3);

%% Berechnung
% Quelle:
% maple_codegen/rotation_rpy_omega.mw
% maple_codegen/codeexport/omega_from_rpy.m

t15 = sin(alpha_s);
t17 = cos(alpha_s);
t18 = sin(beta_s);
t21 = t18 * alphaD_s + gammaD_s;
t19 = cos(beta_s);
t26 = betaD_s * t19;
t35 = t21 * t15 - t17 * t26;
t16 = cos(gamma_s);
t34 = t15 * t16;
t33 = t15 * t18;
t32 = t15 * t19;
t31 = t16 * t17;
t30 = t17 * t18;
t29 = t17 * t19;
t28 = betaD_s * t19 ^ 2;
t27 = betaD_s * t18;
t25 = t19 * alphaD_s;
t24 = t19 * gammaD_s;
t22 = t18 * gammaD_s + alphaD_s;
t20 = t22 * t17;
t14 = sin(gamma_s);
t12 = t15 * t14 - t16 * t30;
t11 = t14 * t30 + t34;
t10 = t14 * t17 + t16 * t33;
t9 = -t14 * t33 + t31;
t8 = -t14 * t24 - t16 * t27;
t7 = t14 * t27 - t16 * t24;
t6 = t15 * t27 - t17 * t25;
t5 = -t15 * t25 - t17 * t27;
t4 = t21 * t31 + (-t22 * t14 + t16 * t26) * t15;
t3 = -t22 * t34 + (-t15 * t26 - t21 * t17) * t14;
t2 = t14 * t20 + t35 * t16;
t1 = -t35 * t14 + t16 * t20;
omega_tilde = [(-t14 * t7 + t16 * t8 + t27) * t19 t10 * t8 - t15 * t28 + t7 * t9 t11 * t7 + t12 * t8 + t17 * t28; t6 * t18 + (-t14 * t3 + t16 * t4) * t19 t4 * t10 + t3 * t9 - t6 * t32 t3 * t11 + t4 * t12 + t6 * t29; t5 * t18 + (-t1 * t14 + t16 * t2) * t19 t1 * t9 + t2 * t10 - t5 * t32 t1 * t11 + t2 * t12 + t5 * t29;];

%% Nachbearbeitung
omega = [omega_tilde(3,2); omega_tilde(1,3); omega_tilde(2,1)];
